simulink model "multilevel"  (R2023a)
settings: Solver=VariableStepAuto  StartTime=0.0  StopTime=1  RelTol=1e-3
libraries: spsMosfetLib x8, spsVoltageMeasurementLib x3, spsDCVoltageSourceLib x2, spspowerguiLib x1, spsSeriesRLCBranchLib x1
settings Model: Creator=burra  LastModifiedBy=vande

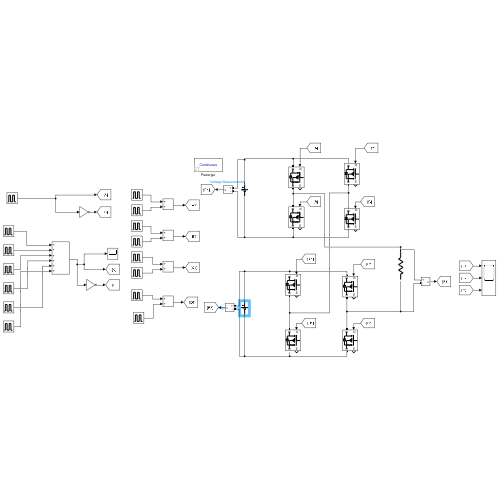
[thumbnail: Simulink's stored preview of the top-level diagram]
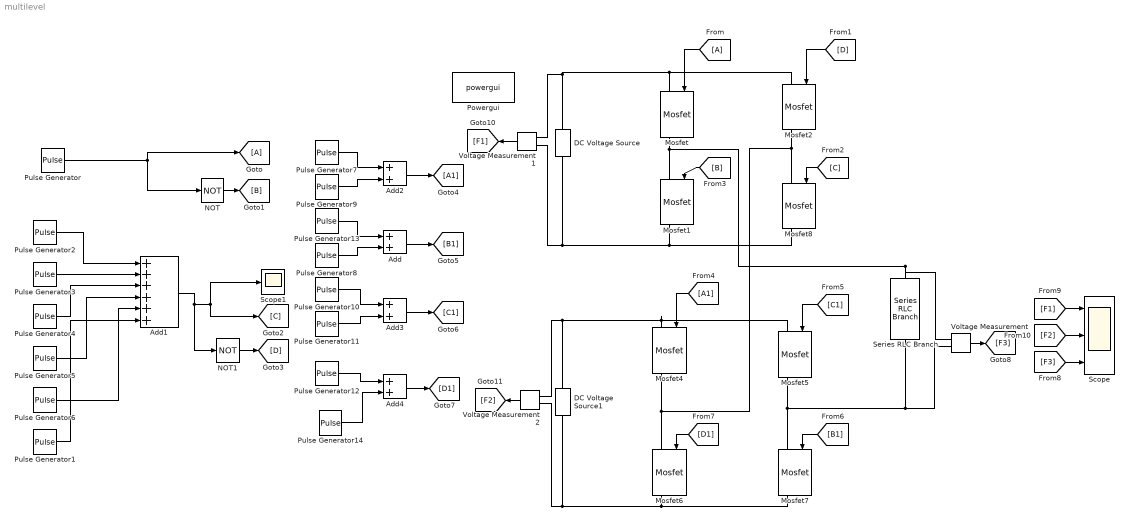
== system multilevel ==
  Add{,2..4} (4 alike) : Sum
  Add1 : Sum  Inputs=++++++
  DC Voltage Source : spsDCVoltageSourceLib/DC Voltage Source  Amplitude=250  Measurements=None
  DC Voltage Source1 : spsDCVoltageSourceLib/DC Voltage Source  Amplitude=500  Measurements=None
  From : From
  Goto : Goto
  Mosfet{,1..2,4..8} (8 alike) : spsMosfetLib/Mosfet  Ron=0.1  Lon=0  Rd=0.01  Vfd=0  IC=0  Rs=1e5  Cs=inf  Measurements=on
  NOT : Logic  Operator=NOT  IconShape=distinctive  AllPortsSameDT=off  OutDataTypeStr=boolean
  NOT1 : Logic  Operator=NOT  IconShape=distinctive  AllPortsSameDT=off  OutDataTypeStr=boolean
  Powergui : spspowerguiLib/powergui  Priority=1  SimulationMode=Continuous  SampleTime=50e-6  frequency=60  Iterations=50  frequencyindice=0  Pbase=100e6  ErrMax=1e-4  UnitsV=kV  UnitsW=MW  buscounter=0  FunctionMessages=off  echomessages=off  EnableUseOfTLC=off  CurrentSourceSwitches=off  DisableSnubberDevices=off  DisableRonSwitches=off  DisableVfSwitches=off  DisplayEquations=off  AutomaticDiscreteSolvers=off  SolverType=Tustin/Backward Euler (TBE)  Interpol=off  ExternalGateDelay=off  methode=off  Ts=100  x0status=blocks  SPID=on  SwTol=0  HookPort=off  NonlinearTolerance=1e-4  nMaxIteration=100  ContinueOnMaxIteration=off  RestoreLinks=warning  ResistiveCurrentMeasurement=off  Frange=[0:2:500]  Ylog=off  Xlog=on  ShowGrid=off  save=off  variable=ZData  structure=0  ZoomFFT=off  StartTime=0.0  cycles=1  DisplayStyle=1  fundamental=60  FreqAxis=off  MaxFrequency=1000  frequencyindicesteady=1  RmsSteady=1  display=off
  Pulse Generator : DiscretePulseGenerator  PulseType=Time based  Period=0.02  PulseWidth=(8/14)*100
  Pulse Generator1 : DiscretePulseGenerator  PulseType=Time based  Period=0.02  PulseWidth=(1/14)*100  PhaseDelay=(13/14)*0.02
  Pulse Generator10 : DiscretePulseGenerator  PulseType=Time based  Period=0.02  PulseWidth=(2/14)*100
  Pulse Generator11 : DiscretePulseGenerator  PulseType=Time based  Period=0.02  PulseWidth=(8/14)*100  PhaseDelay=(5/14)*0.02
  Pulse Generator12 : DiscretePulseGenerator  PulseType=Time based  Period=0.02  PulseWidth=(3/14)*100  PhaseDelay=(9/14)*0.02
  Pulse Generator13 : DiscretePulseGenerator  PulseType=Time based  Period=0.02  PulseWidth=(1/14)*100  PhaseDelay=(13/14)*0.02
  Pulse Generator14 : DiscretePulseGenerator  PulseType=Time based  Period=0.02  PulseWidth=(1/14)*100  PhaseDelay=(13/14)*0.02
  Pulse Generator2 : DiscretePulseGenerator  PulseType=Time based  Period=0.02  PulseWidth=(1/14)*100  PhaseDelay=(1/14)*0.02
  Pulse Generator3 : DiscretePulseGenerator  PulseType=Time based  Period=0.02  PulseWidth=(1/14)*100  PhaseDelay=(3/14)*0.02
  Pulse Generator4 : DiscretePulseGenerator  PulseType=Time based  Period=0.02  PulseWidth=(1/14)*100  PhaseDelay=(5/14)*0.02
  Pulse Generator5 : DiscretePulseGenerator  PulseType=Time based  Period=0.02  PulseWidth=(1/14)*100  PhaseDelay=(9/14)*0.02
  Pulse Generator6 : DiscretePulseGenerator  PulseType=Time based  Period=0.02  PulseWidth=(1/14)*100  PhaseDelay=(11/14)*0.02
  Pulse Generator7 : DiscretePulseGenerator  PulseType=Time based  Period=0.02  PulseWidth=(9/14)*100
  Pulse Generator8 : DiscretePulseGenerator  PulseType=Time based  Period=0.02  PulseWidth=(3/14)*100  PhaseDelay=(2/14)*0.02
  Pulse Generator9 : DiscretePulseGenerator  PulseType=Time based  Period=0.02  PulseWidth=(1/14)*100  PhaseDelay=(12/14)*0.02
  Scope : Scope  NumInputPorts=3
  Scope1 : Scope
  Series RLC Branch : spsSeriesRLCBranchLib/Series RLC Branch  LConnTagsString=__new0  RConnTagsString=__new0  BranchType=R  Resistance=30  Inductance=1e-3  SetiL0=off  InitialCurrent=0  Capacitance=1e-6  Setx0=off  InitialVoltage=0  Measurements=None
  Voltage Measurement : spsVoltageMeasurementLib/Voltage Measurement  PhasorSimulation=off  OutputType=Complex  PSBequivalent=0
  Voltage Measurement1 : spsVoltageMeasurementLib/Voltage Measurement  PhasorSimulation=off  OutputType=Complex  PSBequivalent=0
  Voltage Measurement2 : spsVoltageMeasurementLib/Voltage Measurement  PhasorSimulation=off  OutputType=Complex  PSBequivalent=0
  wires:
  Pulse Generator/1 -> Goto/1, NOT/1
  Pulse Generator6/1 -> Add1/5
  Pulse Generator2/1 -> Add1/1
  Pulse Generator3/1 -> Add1/2
  Pulse Generator4/1 -> Add1/3
  Pulse Generator5/1 -> Add1/4
  Add1/1 -> NOT1/1, Scope1/1, [C]
  Pulse Generator7/1 -> Add2/1
  Pulse Generator9/1 -> Add2/2
  Add2/1 -> [A1]
  Pulse Generator10/1 -> Add3/1
  Pulse Generator11/1 -> Add3/2
  Add3/1 -> [C1]
  NOT/1 -> [B]
  NOT1/1 -> [D]
  [A1] -> Mosfet4/1
  [C1] -> Mosfet5/1
  [D1] -> Mosfet6/1
  [B1] -> Mosfet7/1
  From/1 -> Mosfet/1
  [D] -> Mosfet2/1
  [B] -> Mosfet1/1
  [C] -> Mosfet8/1
  Pulse Generator1/1 -> Add1/6
  Pulse Generator13/1 -> Add/1
  Pulse Generator8/1 -> Add/2
  Add/1 -> [B1]
  Add4/1 -> [D1]
  Pulse Generator12/1 -> Add4/1
  Pulse Generator14/1 -> Add4/2
  Voltage Measurement/1 -> [F3]
  [F1] -> Scope/1
  [F2] -> Scope/2
  [F3] -> Scope/3
  Voltage Measurement2/1 -> [F2]
  Voltage Measurement1/1 -> [F1]
  connections:
  Mosfet/RConn1 -- Mosfet1/LConn1 -- Voltage Measurement/LConn1 -- Series RLC Branch/LConn1
  Mosfet/LConn1 -- DC Voltage Source/RConn1 -- Voltage Measurement1/LConn1 -- Mosfet2/LConn1
  Mosfet1/RConn1 -- DC Voltage Source/LConn1 -- Voltage Measurement1/LConn2 -- Mosfet8/RConn1
  Mosfet4/LConn1 -- DC Voltage Source1/RConn1 -- Voltage Measurement2/LConn1 -- Mosfet5/LConn1
  Mosfet4/RConn1 -- Mosfet2/RConn1 -- Mosfet8/LConn1 -- Mosfet6/LConn1
  Mosfet5/RConn1 -- Series RLC Branch/RConn1 -- Voltage Measurement/LConn2 -- Mosfet7/LConn1
  Mosfet6/RConn1 -- DC Voltage Source1/LConn1 -- Voltage Measurement2/LConn2 -- Mosfet7/RConn1
